simulink subsystem "Potentiometer_2"  (R2024b)
settings: Solver=VariableStepAuto  StartTime=0.0  StopTime=10.0  RelTol=1e-3
undefined symbols (not defined in the file or in its folder): sens, Ts
settings Model: Creator=Federico Bergami  LastModifiedBy=Federico Bergami

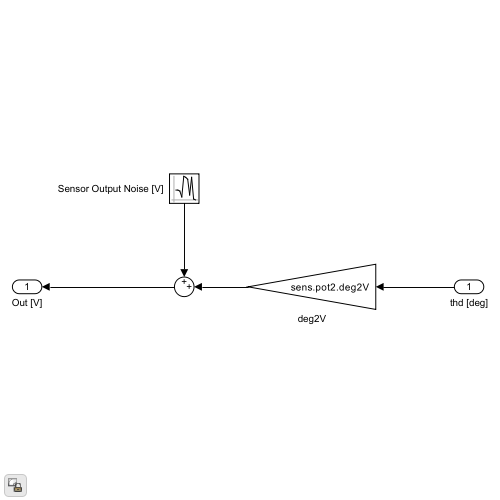
[thumbnail: Simulink's stored preview of the top-level diagram]
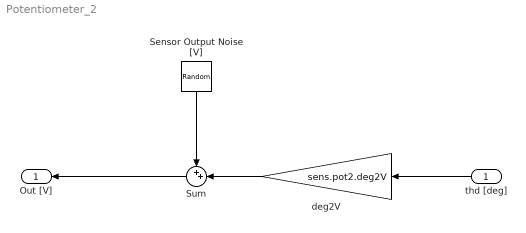
== system Potentiometer_2 ==
  thd [deg] : Inport
  Sensor Output Noise [V] : RandomNumber  Variance=sens.pot2.noise.var  SampleTime=Ts
  Sum : Sum  Inputs=++|
  deg2V : Gain  Gain=sens.pot2.deg2V
  Out [V] : Outport
  wires:
  Sensor Output Noise [V]/1 -> Sum/1
  Sum/1 -> Out [V]/1
  thd [deg]/1 -> deg2V/1
  deg2V/1 -> Sum/2
